simulink model "VDSE_2019b1"  (R2022b)
settings: Solver=ode5  StartTime=0.0  StopTime=T_simulation  FixedStep=simulation_step_time  RelTol=1e-3
values from neighbouring files (symbols this model uses):
  A = 2    [vehicle_parameters_script.m]
  bump_height = 0    [vehicle_parameters_script.m]
  bump_length = 0    [vehicle_parameters_script.m]
  bump_time = 0    [vehicle_parameters_script.m]
  cd = 0.35    [vehicle_parameters_script.m]
  cF = 5000    [vehicle_parameters_script.m]
  clF = -0.15    [vehicle_parameters_script.m]
  clR = -0.20    (= -0.2)    [vehicle_parameters_script.m]
  cp_FA = 30    [vehicle_parameters_script.m]
  cp_RA = 13    [vehicle_parameters_script.m]
  cR = 5000    [vehicle_parameters_script.m]
  ctF = tireF.VERTICAL_DAMPING    [vehicle_parameters_script.m]
  ctR = tireR.VERTICAL_DAMPING    [vehicle_parameters_script.m]
  enableDriverControl = 1    [vehicle_parameters_script.m]
  enableLongDynamics = 1    [vehicle_parameters_script.m]
  enablePowertrain = 1    [vehicle_parameters_script.m]
  g = 9.806    [vehicle_parameters_script.m]
  Gear_numbers = [1 2 3 4 5 6]    [vehicle_parameters_script.m]
  GR = [2.9 1.8 1.3 1 0.85 0.75]    [vehicle_parameters_script.m]
  hcog = 0.441    [vehicle_parameters_script.m]
  hpc = 0.0    (= 0)    [vehicle_parameters_script.m]
  hrcF = 0.3    [vehicle_parameters_script.m]
  hrcg = (hrcF*lR+hrcR*lF)/(lF+lR)    (= 0.25108)    [vehicle_parameters_script.m]
  hrcR = 0.2    [vehicle_parameters_script.m]
  huFcog = 0.32    [vehicle_parameters_script.m]
  huRcog = 0.32    [vehicle_parameters_script.m]
  i1 = 11.42    [vehicle_parameters_script.m]
  i2 = 3.727    [vehicle_parameters_script.m]
  initial_gear = 1    [vehicle_parameters_script.m]
  JwF = 2.45    [vehicle_parameters_script.m]
  JwR = 2.45    [vehicle_parameters_script.m]
  Jx = 4.12    [vehicle_parameters_script.m]
  Jy = 109.16    [vehicle_parameters_script.m]
  Jz = 105.13    [vehicle_parameters_script.m]
  kF = 40000    [vehicle_parameters_script.m]
  kR = 35000    [vehicle_parameters_script.m]
  kRF = 0    [vehicle_parameters_script.m]
  kRR = 0    [vehicle_parameters_script.m]
  ktF = tireF.VERTICAL_STIFFNESS    [vehicle_parameters_script.m]
  ktR = tireR.VERTICAL_STIFFNESS    [vehicle_parameters_script.m]
  lF = 1.223    [vehicle_parameters_script.m]
  lR = l-lF    (= 1.277)    [vehicle_parameters_script.m]
  m = 340    [vehicle_parameters_script.m]
  max_pressure = 1000    [vehicle_parameters_script.m]
  maxrpm = 4000    [vehicle_parameters_script.m]
  mF = 45    [vehicle_parameters_script.m]
  minrpm = 1500    [vehicle_parameters_script.m]
  mR = 50    [vehicle_parameters_script.m]
  output_samping_time = 0.001    [vehicle_parameters_script.m]
  phi0 = 0    [vehicle_parameters_script.m]
  phi_dot0 = 0    [vehicle_parameters_script.m]
  psi0 = 0    [vehicle_parameters_script.m]
  psi_dot0 = 0    [vehicle_parameters_script.m]
  RearRatio = 1    [vehicle_parameters_script.m]
  requested_speed = 120/3.6    (= 33.3333333333)    [vehicle_parameters_script.m]
  rF = tireF.UNLOADED_RADIUS    [vehicle_parameters_script.m]
  rho = 1.2    [vehicle_parameters_script.m]
  rR = tireR.UNLOADED_RADIUS    [vehicle_parameters_script.m]
  steer_ratio = 13.25    [vehicle_parameters_script.m]
  TFL = 0    [vehicle_parameters_script.m]
  TFR = 0    [vehicle_parameters_script.m]
  theta0 = 0    [vehicle_parameters_script.m]
  theta_dot0 = 0    [vehicle_parameters_script.m]
  TRL = 0    [vehicle_parameters_script.m]
  TRR = 0    [vehicle_parameters_script.m]
  Vx0 = 0.01/3.6    (= 0.00277777777778)    [vehicle_parameters_script.m]
  Vy0 = 0    [vehicle_parameters_script.m]
  Vz0 = 0    [vehicle_parameters_script.m]
  wF = 1.578    [vehicle_parameters_script.m]
  wR = 1.544    [vehicle_parameters_script.m]
  x0 = 0    [vehicle_parameters_script.m]
  xcog_overall = (2*mR*xR+2*xF*mF+m*xs)/(m+2*mF+2*mR)    (= 1.25626415094)    [vehicle_parameters_script.m]
  y0 = 0    [vehicle_parameters_script.m]
  z0 = 0    [vehicle_parameters_script.m]
  zFL0 = 0    [vehicle_parameters_script.m]
  zFL_dot0 = 0    [vehicle_parameters_script.m]
  zFR0 = 0    [vehicle_parameters_script.m]
  zFR_dot0 = 0    [vehicle_parameters_script.m]
  zRL0 = 0    [vehicle_parameters_script.m]
  zRL_dot0 = 0    [vehicle_parameters_script.m]
  zRR0 = 0    [vehicle_parameters_script.m]
  zRR_dot0 = 0    [vehicle_parameters_script.m]
undefined symbols (not defined in the file or in its folder): Bxf, Bxr, Byf, Byr, Cxf, Cxr, Cyf, Cyr, DiscIntNeverNeededParam, Dxf, Dxr, Dyf, Dyr, exf, exr, eyf, eyr, FNOMINf, FNOMINr, Ldwf, Ldwr, PCX1f, PCX1r, PCY1f, PCY1r, PDX1f, PDX1r, PDX2f, PDX2r, PDY1f, PDY1r, PDY2f, PDY2r, PDY3f, PDY3r, PEX1f, PEX1r, PEX2f, PEX2r, PEX3f, PEX3r, PEX4f, PEX4r, PEY1f, PEY1r, PEY2f, PEY2r, PEY3f, PEY3r, PEY4f, PEY4r, PHX1f, PHX1r, PHX2f, PHX2r, PHY1f, PHY1r, PHY2f, PHY2r, PHY3f ... (+147)
libraries: simulink x55, mfeval_LIB x4, slpidlib x1
(part 7 of 7)

== matlab function VDSE_2019b1/14-DOF VEHICLE MODEL/WHEEL ASSEMBLY/WHEEL ASSEMBLY PACEIJKA/TIRE VELOCITIES ==
  data: deltaFL input; VFLx output; VFLy output; VFRx output; VFRy output; VRLx output; VRLy output; VRRx output; deltaFR input; deltaRL input; deltaRR input; V input; beta input; psidot input; VRRy output; lF input; lR input; wFL input; wFR input; wRL input; wRR input
function [VFLx, VFLy, VFRx, VFRy, VRLx, VRLy, VRRx, VRRy] = ConversiontoCorners(deltaFL,deltaFR,deltaRL,deltaRR,...
    V, beta, psidot,  lF, lR, wFL, wFR, wRL, wRR)
% Geometric calcs
lFL = sqrt(lF^2+wFL^2); gammaFL = atan2(wFL,lF);
lFR = sqrt(lF^2+wFR^2); gammaFR = atan2(wFR,lF);
lRL = sqrt(lR^2+wRL^2); gammaRL = atan2(wRL,lR);
lRR = sqrt(lR^2+wRR^2); gammaRR = atan2(wRR,lR);

% Tire Velocities
VFLx = V*cos(deltaFL - beta) - psidot*lFL*sin(gammaFL - deltaFL);
VFLy = - V*sin(deltaFL - beta) + psidot*lFL*cos(gammaFL - deltaFL);
VFRx = V*cos(deltaFR - beta) + psidot*lFR*sin(gammaFR + deltaFR);
VFRy = - V*sin(deltaFR - beta) + psidot*lFR*cos(gammaFR + deltaFR);
VRLx = V*cos(deltaRL - beta) - psidot*lRL*sin(gammaRL + deltaRL);
VRLy = -V*sin(deltaRL - beta) - psidot*lRL*cos(gammaRL + deltaRL);
VRRx = V*cos(deltaRR - beta) + psidot*lRR*sin(gammaRR - deltaRR);
VRRy = -V*sin(deltaRR - beta) - psidot*lRR*cos(gammaRR - deltaRR);
end

== matlab function VDSE_2019b1/14-DOF VEHICLE MODEL/EQUATIONS OF MOTION FOR CHASSIS/Lateral Dynamics/LATERAL DYNAMICS ==
  data: deltaFL input; ay output; fFLx input; fFLy input; deltaFR input; fFRx input; fFRy input; deltaRL input; fRLx input; fRLy input; deltaRR input; fRRx input; fRRy input; mFLy input; mFRy input; mRLy input; mRRy input; Vx input; psi_dot input; phi_dot input; Vz input; m input; mF input; mR input; Vy_dot output; rF input; rR input
function [ay, Vy_dot] = lateral_dynamics(deltaFL, fFLx, fFLy, deltaFR, fFRx, fFRy, deltaRL, fRLx, fRLy, deltaRR, fRRx, fRRy,...
    mFLy, mFRy, mRLy, mRRy, Vx, psi_dot, phi_dot, Vz, m, mF, mR, rF, rR)
% Parameters:
% m = sprung mass [kg]
% mF = half front unsprung mass [kg]
% mR = half rear unsprung mass [kg]
%
% Annotations:
% fijx, fijy = force at the tire frame [N]
% mijy = rolling moment at the tire frame [Nm]
% ay = overall lateral acceleration [m/s^2]
% Vy_dot = lateral acceleration excluding tangential terms [m/s^2]
% phi_dot = roll angular velocity [rad/s]
% psi_dot = yaw angular velocity [rad/s]
% Vz = vertical sprung mass velocity [m/s]
% Vx = longitudinal vehicle's velocity [m/s]
% deltaFL = FL wheel's steering angle [rad]
% deltaFR = FR wheel's steering angle [rad]
% deltaRL = RL wheel's steering angle [rad]
% deltaRR = RR wheel's steering angle [rad]
%
% i: F, R = Front, Rear
% j: R, L = Right, Left

% Projection in the vehicle frame:
fFLy_vehicle=fFLy*cos(deltaFL)+fFLx*sin(deltaFL);
fFRy_vehicle=fFRy*cos(deltaFR)+fFRx*sin(deltaFR);
fRLy_vehicle=fRLy*cos(deltaRL)+fRLx*sin(deltaRL);
fRRy_vehicle=fRRy*cos(deltaRR)+fRRx*sin(deltaRR);

% Calculation of overall lateral acceleration:
ay = (fFLy_vehicle+fFRy_vehicle+fRLy_vehicle+fRRy_vehicle+mFLy/rF*sin(deltaFL)+...
    mFRy/rF*sin(deltaFR)+mRLy/rR*sin(deltaRL)+mRRy/rR*sin(deltaRR))/(m+2*mF+2*mR);

% Calculation of vehicle's lateral acceleration excluding tangential terms:
Vy_dot = ay - Vx*psi_dot + phi_dot*Vz ;


end

== matlab function VDSE_2019b1/14-DOF VEHICLE MODEL/EQUATIONS OF MOTION FOR CHASSIS/Yaw Dynamics/YAW DYNAMICS ==
  data: deltaFL input; psi_dot_dot output; fFLx input; fFLy input; deltaFR input; fFRx input; fFRy input; deltaRL input; fRLx input; fRLy input; deltaRR input; fRRx input; fRRy input; ay input; mFLz input; mFRz input; mRLz input; mRRz input; wF input; wR input; mF input; mR input; lF input; lR input; Jz input
function psi_dot_dot = yaw_dynamics(deltaFL, fFLx, fFLy, deltaFR, fFRx, fFRy, deltaRL, fRLx, fRLy, deltaRR, fRRx, fRRy, ...
    ay, mFLz, mFRz, mRLz, mRRz, wF, wR, mF, mR, lF, lR, Jz)

% Parameters:
% m = sprung mass [kg]
% mF = half front unsprung mass [kg]
% mR = half rear unsprung mass [kg]
% lF = front wheel base [m]
% lR = rear wheel base [m]
% wF = front trackwidth [m]
% wR = rear trackwidth [m]
% Jz = yaw moment of inertia [kgm^2]
%
% Annotations:
% fijx, fijy = force at the tire frame [N]
% mijz = overturning moment at the tire frame [Nm]
% psi_dot_dot = yaw angular acceleration [rad/s]
% ay = vehicle's overall lateral acceleration [m/s^2]
% deltaFL = FL wheel's steering angle [rad]
% deltaFR = FR wheel's steering angle [rad]
% deltaRL = RL wheel's steering angle [rad]
% deltaRR = RR wheel's steering angle [rad]
%
% i: F, R = Front, Rear
% j: R, L = Right, Left

% Summation of moments:
sum = (fFLy*cos(deltaFL)+fFRy*cos(deltaFR)+fFLx*sin(deltaFL)+fFRx*sin(deltaFR))*lF...
    -(fRLy*cos(deltaRL)+fRRy*cos(deltaRR)+fRLx*sin(deltaRL)+fRRx*sin(deltaRR))*lR...
    +fFLy*sin(deltaFL)*wF/2-fFLx*cos(deltaFL)*wF/2+fRLy*sin(deltaRL)*wR/2-fRLx*cos(deltaRL)*wR/2 ...
    -fFRy*sin(deltaFR)*wF/2+fFRx*cos(deltaFR)*wF/2-fRRy*sin(deltaRR)*wR/2+fRRx*cos(deltaRR)*wR/2 ...
    +mFLz+mFRz+mRLz+mRRz...
    +(2*mR*lR-2*mF*lF)*ay;

% Yaw angular acceleration calculation:
psi_dot_dot = sum/Jz;
end

== matlab function VDSE_2019b1/DRIVER CONTROL/MATLAB Function ==
  data: brake input; Vx input; Brake_Cmd output
function Brake_Cmd = check(brake, Vx)
Brake_Cmd = brake;
if Vx<0
    Brake_Cmd = 0;
end

end

== matlab function VDSE_2019b1/14-DOF VEHICLE MODEL/SUSPENSION/Load Transfer/Tire lift from the ground check ==
  data: FLz_Overall input; FLz output; FRz_Overall input; RLz_Overall input; RRz_Overall input; ax input; ay input; FRz output; RLz output; RRz output; time input; trackwidth input; wheelbase input
function [FLz,FRz,RLz,RRz] = LiftFromGroundCheck(FLz_Overall,FRz_Overall,RLz_Overall,RRz_Overall,ax,ay,time, trackwidth, wheelbase)
                
if(time<1e-3)
    FLz=FLz_Overall;
    FRz=FRz_Overall;
    RLz=RLz_Overall;
    RRz=RRz_Overall;
    return
end
ax=abs(ax/wheelbase);
ay=abs(ay/trackwidth);
prop_lat=ay/(ax+ay);
prop_long=ax/(ax+ay);
FLz=FLz_Overall;
FRz=FRz_Overall;
RLz=RLz_Overall;
RRz=RRz_Overall;
fz_out = [FLz FRz RLz RRz];

while(min(fz_out)<0)
    [i,j] = find(fz_out <0);
    if(~isempty(find(j == 1)))
        if(fz_out(2) ==0)
            fz_out(4) = fz_out(4) + prop_lat*fz_out(1);
            fz_out(3) = fz_out(3) + prop_long*fz_out(1);
            fz_out(1) = 0;
        elseif (fz_out(3) ==0)
            fz_out(2) = fz_out(2) + prop_lat*fz_out(1);
            fz_out(4) = fz_out(4) + prop_long*fz_out(1);
            fz_out(1) = 0;
        else
        fz_out(2) = fz_out(2) + prop_lat*fz_out(1); %FRz=FRz_Overall+prop_lat*FLz_Overall;
        fz_out(3) = fz_out(3) + prop_long*fz_out(1); %RLz=RLz_Overall+prop_long*FLz_Overall;
        fz_out(1) = 0;
        end
    end
    
    if(~isempty(find(j == 2)))
        if(fz_out(1) ==0)
            fz_out(4) = fz_out(4) + prop_long*fz_out(2);
            fz_out(3) = fz_out(1) + prop_lat*fz_out(2);
            fz_out(2) = 0;
        elseif (fz_out(4) ==0)
            fz_out(1) = fz_out(1) + prop_lat*fz_out(2);
            fz_out(3) = fz_out(3) + prop_long*fz_out(2);
            fz_out(2) = 0;
        else
        fz_out(1) = fz_out(1) + prop_lat*fz_out(2); %FLz=FLz_Overall+prop_lat*FRz_Overall;
        fz_out(4) = fz_out(4) + prop_long*fz_out(2); %RRz=RRz_Overall+prop_long*FRz_Overall;
        fz_out(2) = 0;
        end
    end
    
    if(~isempty(find(j == 3)))
        if(fz_out(1) ==0)
            fz_out(4) = fz_out(4) + prop_lat*fz_out(3);
            fz_out(2) = fz_out(2) + prop_long*fz_out(3);
            fz_out(3) = 0;
        elseif (fz_out(4) ==0)
            fz_out(1) = fz_out(1) + prop_long*fz_out(3);
            fz_out(2) = fz_out(2) + prop_lat*fz_out(3);
            fz_out(3) = 0;
        else        
        fz_out(4) = fz_out(4) + prop_lat*fz_out(3);%RRz=RRz_Overall+prop_lat*RLz_Overall;
        fz_out(1) = fz_out(1) + prop_long*fz_out(3);%FLz=FLz_Overall+prop_long*RLz_Overall;
        fz_out(3) = 0;
        end
    end
    
    if(~isempty(find(j == 4)))
        if(fz_out(3) == 0)
            fz_out(2) = fz_out(2) +  prop_long*fz_out(4);
            fz_out(1) = fz_out(1) + prop_lat*fz_out(4);
            fz_out(4) = 0;
        elseif (fz_out(2) == 0)
            fz_out(3) = fz_out(3) + prop_lat*fz_out(2);
            fz_out(1) = fz_out(1) + prop_long*fz_out(4);
            fz_out(4) = 0;
        else        
        fz_out(3) =  fz_out(3) + prop_lat*fz_out(4);%RLz=RLz_Overall+prop_lat*RRz_Overall;
        fz_out(2) = fz_out(2) + prop_long*fz_out(4);%FRz=FRz_Overall+prop_long*RRz_Overall;
        fz_out(4) = 0;
        end
    end

end
FLz = fz_out(1);FRz = fz_out(2);RLz = fz_out(3);RRz = fz_out(4);
end
